simulink model "Drone_example_2017a"  (R2017a)
settings: Solver=VariableStepAuto  StartTime=0.0  StopTime=inf  RelTol=1e-3
model workspace: external: MATLAB File /Users/davekooijman/Documents/vrep-matlab-interface/Initialize_visualisation.m (data not in the file)
values from neighbouring files (symbols this model uses):
  dt_hl = 1/20    (= 0.05)    [Initialize_visualisation.m]
  dt_ll = 1/200    (= 0.005)    [Initialize_visualisation.m]
  dt_visual = 1/20    (= 0.05)    [Initialize_visualisation.m]
  g = 9.81    [Initialize_visualisation.m]
  mass = 1.05    [Initialize_visualisation.m]
libraries: sharedtransform x1, shared6dof x1
settings Model: Creator=davekooijman  LastModifiedBy=davekooijman

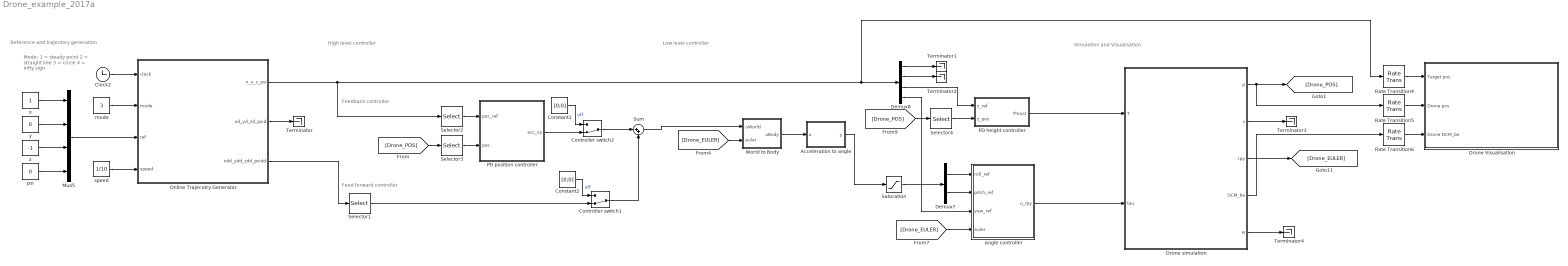
== system Drone_example_2017a ==
  note: Reference and trajectory generation
  note: High level controller
  note: Low level controller
  note: Feed forward controller
  note: Feedback controller
  note: Mode:
      | 1 = steady point
      | 2 = straight line
      | 3 = circle
      | 4 = infty sign
  note: Simulation and Visualisation
  Acceleration to angle : MATLAB Function  TreatAsAtomicUnit=on
  Angle controller : MATLAB Function
  Clock2 : Clock
  Constant1 : Constant  Value=[0;0]
  Constant2 : Constant  Value=[0;0]
  Controller switch1 : ManualSwitch  CurrentSetting=0
  Controller switch2 : ManualSwitch  CurrentSetting=0
  Demux7 : Demux  Outputs=2
  Demux8 : Demux
  Drone Visualisation : Subsystem  TreatAsAtomicUnit=on  SystemSampleTime=dt_visual
      settings: MinAlgLoopOccurrences=on
      mask Display: image('Drone_visualisation.png');
  Drone simulation : Subsystem
  Mux5 : Mux
  Online Trajecotry Generator : MATLAB Function  TreatAsAtomicUnit=on  SystemSampleTime=dt_ll
  PD height controller : Subsystem
  "PD position controller " : MATLAB Function  TreatAsAtomicUnit=on  SystemSampleTime=dt_hl
  Rate Transition4 : RateTransition
  Rate Transition5 : RateTransition
  Rate Transition6 : RateTransition
  Saturation : Saturate  UpperLimit=0.471  LowerLimit=-0.471
  Selector1 : Selector  InputPortWidth=4  IndexOptions=Index vector (dialog)  Indices=[1 2]  OutputSizes=1
  Selector2 : Selector  InputPortWidth=4  IndexOptions=Index vector (dialog)  Indices=[1 2]  OutputSizes=1
  Selector3 : Selector  InputPortWidth=3  IndexOptions=Index vector (dialog)  Indices=[1 2]  OutputSizes=1
  Selector4 : Selector  InputPortWidth=3  IndexOptions=Index vector (dialog)  Indices=[3]  OutputSizes=1
  Sum : Sum  Inputs=|++
  Terminator{,1..4} (5 alike) : Terminator
  World to Body : MATLAB Function  TreatAsAtomicUnit=on
  mode : Constant  Value=3
  psi : Constant  Value=0
  speed : Constant  Value=1/10
  x : Constant
  y : Constant  Value=0
  z : Constant  Value=-1
  wires:
  Constant2/1 -> Controller switch1/1  "off"
  Online Trajecotry Generator/3(xdd_ydd_zdd_psidd) -> Selector1/1
  Demux7/1 -> Angle controller/1(roll_ref)
  Selector2/1 -> "PD position controller "/1(pos_ref)
  Controller switch1/1 -> Sum/2
  Selector4/1 -> PD height controller/2(z_pos)
  Constant1/1 -> Controller switch2/1  "off"
  z/1 -> Mux5/3
  Demux7/2 -> Angle controller/2(pitch_ref)
  Demux8/4 -> Angle controller/3(yaw_ref)
  Demux8/3 -> PD height controller/1(z_ref)
  mode/1 -> Online Trajecotry Generator/2(mode)
  Selector1/1 -> Controller switch1/2
  [Drone_EULER] -> Angle controller/4(euler)
  Acceleration to angle/1(y) -> Saturation/1
  [Drone_EULER] -> World to Body/2(euler)
  psi/1 -> Mux5/4
  Saturation/1 -> Demux7/1
  y/1 -> Mux5/2
  World to Body/1(uBody) -> Acceleration to angle/1(u)
  Controller switch2/1 -> Sum/1
  Online Trajecotry Generator/2(xd_yd_zd_psid) -> Terminator/1
  Mux5/1 -> Online Trajecotry Generator/3(ref)
  x/1 -> Mux5/1
  "PD position controller "/1(acc_xy) -> Controller switch2/2
  [Drone_POS] -> Selector4/1
  speed/1 -> Online Trajecotry Generator/4(speed)
  Selector3/1 -> "PD position controller "/2(pos)
  [Drone_POS] -> Selector3/1
  Clock2/1 -> Online Trajecotry Generator/1(clock)
  Rate Transition4/1 -> Drone Visualisation/1(Target pos)
  Drone simulation/5(w) -> Terminator4/1
  Angle controller/1(u_rpy) -> Drone simulation/2(tau)
  Rate Transition5/1 -> Drone Visualisation/2(Drone pos)
  Rate Transition6/1 -> Drone Visualisation/3("Drone DCM_be ")
  Drone simulation/1(p) -> [Drone_POS], Rate Transition5/1
  Online Trajecotry Generator/1(x_y_z_psi) -> Rate Transition4/1, Demux8/1, Selector2/1
  PD height controller/1(Thrust) -> Drone simulation/1(T)
  Drone simulation/2(v) -> Terminator3/1
  Drone simulation/3(rpy) -> [Drone_EULER]
  Drone simulation/4(DCM_be) -> Rate Transition6/1
  Demux8/1 -> Terminator1/1
  Demux8/2 -> Terminator2/1
  Sum/1 -> World to Body/1(uWorld)

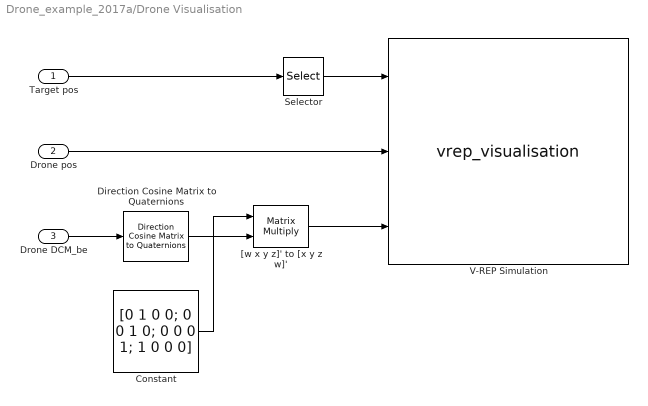
== system Drone_example_2017a/Drone Visualisation ==
  Target pos : Inport
  Drone pos : Inport  Port=2
  "Drone DCM_be " : Inport  Port=3
  Constant : Constant  Value=[0 1 0 0; 0 0 1 0; 0 0 0 1; 1 0 0 0]
  Direction Cosine Matrix to Quaternions : sharedtransform/Direction Cosine Matrix  to Quaternions
      settings: SourceProductName=Aerospace Blockset  SourceProductBaseCode=AE
  Selector : Selector  InputPortWidth=4  IndexOptions=Index vector (dialog)  Indices=[1:3]  OutputSizes=1
  V-REP Simulation : M-S-Function  FunctionName=vrep_visualisation  Parameters=dt_visual, '127.0.0.1'
      mask Display: image('Drone.png');
  "[w x y z]' to [x y z w]'" : Product  Multiplication=Matrix(*)
  wires:
  Selector/1 -> V-REP Simulation/1
  Target pos/1 -> Selector/1
  Drone pos/1 -> V-REP Simulation/2
  "[w x y z]' to [x y z w]'"/1 -> V-REP Simulation/3
  Constant/1 -> "[w x y z]' to [x y z w]'"/1
  "Drone DCM_be "/1 -> Direction Cosine Matrix to Quaternions/1
  Direction Cosine Matrix to Quaternions/1 -> "[w x y z]' to [x y z w]'"/2

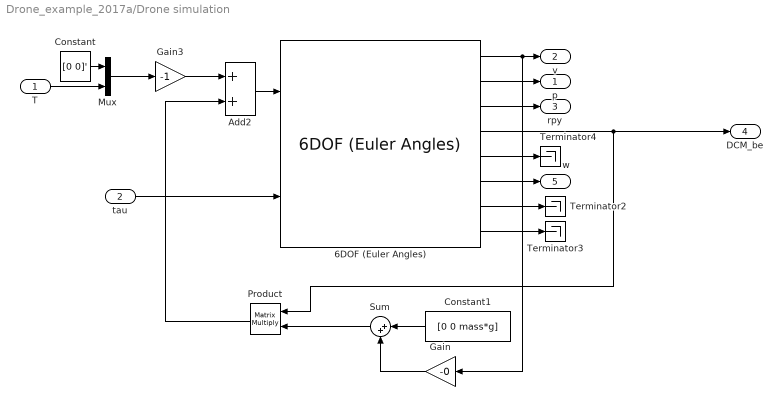
== system Drone_example_2017a/Drone simulation ==
  T : Inport
  tau : Inport  Port=2
  6DOF (Euler Angles) : shared6dof/6DOF (Euler Angles)  units=Metric (MKS)  mtype=Fixed  rep=Euler Angles  xme_0=[0 0 -1]'  Vm_0=[0 0 0]  eul_0=[0 0 0]  pm_0=[0 0 0]  mass_0=mass  mass_e=0.5  mass_f=2.0  inertia=MomInertia  inertia_e=eye(3)  inertia_f=2*eye(3)  k_quat=1.0  vre_flag=on  abi_flag=off
      settings: SourceProductBaseCode=AE
  Add2 : Sum
  Constant : Constant  Value=[0 0]'
  Constant1 : Constant  Value=[0 0 mass*g]
  Gain : Gain  Gain=-0
  Gain3 : Gain  Gain=-1
  Mux : Mux  Inputs=2
  Product : Product  Multiplication=Matrix(*)
  Sum : Sum  Inputs=|++
  Terminator2 : Terminator
  Terminator3 : Terminator
  Terminator4 : Terminator
  p : Outport
  v : Outport  Port=2
  rpy : Outport  Port=3
  DCM_be : Outport  Port=4
  w : Outport  Port=5
  wires:
  6DOF (Euler Angles)/8 -> Terminator3/1
  Product/1 -> Add2/2
  6DOF (Euler Angles)/7 -> Terminator2/1
  Add2/1 -> 6DOF (Euler Angles)/1
  6DOF (Euler Angles)/1 -> Gain/1, v/1
  6DOF (Euler Angles)/2 -> p/1
  Constant/1 -> Mux/1
  Gain3/1 -> Add2/1
  6DOF (Euler Angles)/3 -> rpy/1
  6DOF (Euler Angles)/5 -> Terminator4/1
  Mux/1 -> Gain3/1
  6DOF (Euler Angles)/6 -> w/1
  T/1 -> Mux/2
  tau/1 -> 6DOF (Euler Angles)/2
  6DOF (Euler Angles)/4 -> DCM_be/1, Product/1
  Constant1/1 -> Sum/1
  Sum/1 -> Product/2
  Gain/1 -> Sum/2

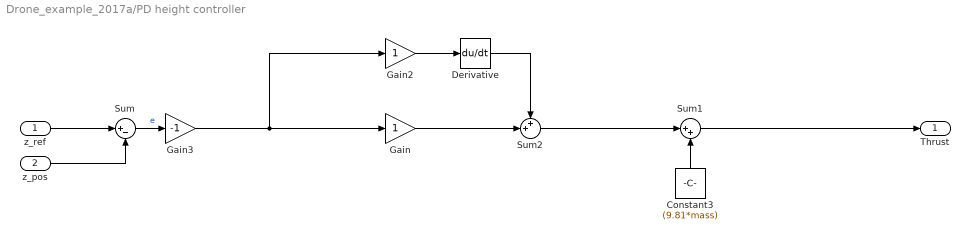
== system Drone_example_2017a/PD height controller ==
  z_ref : Inport
  z_pos : Inport  Port=2
  Constant3 : Constant  Value=(9.81*mass)
  Derivative : Derivative
  Gain : Gain
  Gain2 : Gain
  Gain3 : Gain  Gain=-1
  Sum : Sum  Inputs=|+-
  Sum1 : Sum  Inputs=|++
  Sum2 : Sum  Inputs=++|
  Thrust : Outport
  wires:
  Constant3/1 -> Sum1/2
  Sum/1 -> Gain3/1  "e"
  z_ref/1 -> Sum/1
  z_pos/1 -> Sum/2
  Sum1/1 -> Thrust/1
  Gain2/1 -> Derivative/1
  Sum2/1 -> Sum1/1
  Gain/1 -> Sum2/2
  Derivative/1 -> Sum2/1
  Gain3/1 -> Gain2/1, Gain/1

== matlab function Drone_example_2017a/PD position controller  ==
  settings: updateMethod=DISCRETE
  data: pos_ref input; acc_xy output; pos input; dt_hl parameter
function acc_xy  = fcn(pos_ref, pos, dt_hl)
persistent prev_err
err = pos_ref-pos;
if isempty(prev_err)
    prev_err = err;
end
kp = 5;
kd = 1;
acc_xy = kp*err + kd*(err-prev_err)/dt_hl;
prev_err = err;

== matlab function Drone_example_2017a/Angle controller ==
  settings: updateMethod=DISCRETE
  data: roll_ref input; u_rpy output; pitch_ref input; yaw_ref input; euler input; dt_ll parameter
function u_rpy = fcn(roll_ref, pitch_ref, yaw_ref, euler, dt_ll)
persistent pref_roll_err pref_pitch_err pref_yaw_err
roll = euler(1);
pitch = euler(2);
yaw = euler(3);

roll_err = (roll_ref-roll);
pitch_err = (pitch_ref-pitch);
yaw_err = (yaw_ref-yaw);

if isempty(pref_roll_err)
    pref_roll_err = roll_err;
end
if isempty(pref_pitch_err)
    pref_pitch_err = pitch_err;
end
if isempty(pref_yaw_err)
    pref_yaw_err = yaw_err;
end

kp = 0.5;
kd = 0.025;

u_roll = kp*roll_err + kd*(roll_err-pref_roll_err)/dt_ll;
u_pitch = kp*pitch_err + kd*(pitch_err-pref_pitch_err)/dt_ll;
u_yaw = 0.002*yaw_err + 0.01*(yaw_err-pref_yaw_err)/dt_ll;

%saturate u_yaw
max_u_yaw = 0.02;
if abs(u_yaw) > max_u_yaw
    u_yaw = sign(u_yaw)*max_u_yaw;
end

u_rpy = [u_roll; u_pitch; u_yaw];
pref_roll_err = roll_err;
pref_pitch_err = pitch_err;
pref_yaw_err = yaw_err;

== matlab function Drone_example_2017a/Online Trajecotry Generator ==
  data: clock input; mode input; ref input; x_y_z_psi output; dt_hl parameter; speed input; xd_yd_zd_psid output; xdd_ydd_zdd_psidd output
%%%%%%%%%%%%%%%%%%%%%%%%%%%%%%%%%%%%%%%%%%%%%%%%%%%%%%%%%%%%%%%%%%%%%%%%%%%
%
% File: Online Trajecotry Generator
%
% REMARKS
%
% created with MATLAB ver.: 9.3.0.713579 (R2017b) on Mac OS X  Version: 10.13.2 Build: 17C76a
%
% created by: Dave Kooijman
% DATE: 22-Nov-2017
%
%%%%%%%%%%%%%%%%%%%%%%%%%%%%%%%%%%%%%%%%%%%%%%%%%%%%%%%%%%%%%%%%%%%%%%%%%%%
function [x_y_z_psi, xd_yd_zd_psid, xdd_ydd_zdd_psidd]= fcn(clock, mode, ref, dt_hl, speed)
% opt = option
% 1 = static point
% 2 = straight line
% 3 = circle


%define variables;
x = 0;
y = 0;
z = 0;
psi = 0;
x_dot = 0;
y_dot = 0;
z_dot = 0;
psi_dot = 0;
x_ddot = 0;
y_ddot = 0;
z_ddot = 0;
psi_ddot = 0;

%overwrite variables

switch mode
    case 1
        x = ref(1);
        y = ref(2);
        z = ref(3);
        psi = ref(4);
        x_dot = 0;
        y_dot = 0;
        z_dot = 0;
        psi_dot = 0;
        x_ddot = 0;
        y_ddot = 0;
        z_ddot = 0;
        psi_ddot = 0;
        
    case 2
        fr = speed*2*pi;
        x = sin(clock*fr);
        y = ref(2);
        z = ref(3);
        psi = ref(4);
        x_dot = cos(clock*fr)*fr;
        y_dot = 0;
        z_dot = 0;
        psi_dot = 0;
        x_ddot = -sin(clock*fr)*fr^2;
        y_ddot= 0;
        z_ddot = 0;
        psi_ddot = 0;
        
    case 3
        fr = speed*2*pi;
        x = sin(clock*fr);
        y = cos(clock*fr);
        z = ref(3);
        psi = ref(4);
        x_dot = cos(clock*fr)*fr;
        y_dot = -sin(clock*fr)*fr;
        z_dot = 0;
        psi_dot_vec = 0;
        x_ddot = -sin(clock*fr)*fr^2;
        y_ddot = cos(clock*fr)*fr^2;
        z_ddot = 0;
        psi_ddot = 0;
        
    otherwise
        
end

x_y_z_psi = [x;y;z;psi];
xd_yd_zd_psid = [x_dot; y_dot; z_dot; psi_dot];
xdd_ydd_zdd_psidd = [x_ddot; y_ddot; z_ddot; psi_ddot];
end

== matlab function Drone_example_2017a/Acceleration to angle ==
  data: u input; y output
function y = fcn(u)
y = atan(u/(9.81));

== matlab function Drone_example_2017a/World to Body ==
  data: uWorld input; uBody output size=2,1; euler input
function uBody = fcn(uWorld, euler)
uBody = [0;0];
phi = euler(1);
theta = euler(2);
psi = euler(3);

Rx = [1 0 0; 0 cos(phi) -sin(phi); 0 sin(phi) cos(phi)];
Ry = [cos(theta) 0 sin(theta); 0 1 0; -sin(theta) 0 cos(theta)];
Rz = [cos(psi) -sin(psi) 0; sin(psi) cos(psi) 0; 0 0 1];
R = Rx*Ry*Rz; %VREP-uses Rx*Ry*Rz euler rotations


body = R\[uWorld(2); -uWorld(1); 0];
uBody = [body(1); body(2)];
